simulink library "HVPS_AC120V_sfun_xk"  (R2022b)
settings: Solver=VariableStepAuto  StartTime=0.0  StopTime=10.0  RelTol=1e-3
Description:
  | Created by MapleSim.
settings Model: Creator=MapleSim  LastModifiedBy=BEDNASA

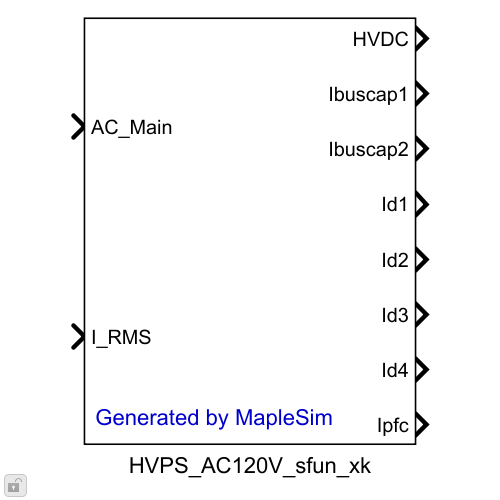
[thumbnail: Simulink's stored preview of the top-level diagram]
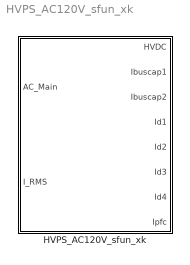
== system HVPS_AC120V_sfun_xk ==
  HVPS_AC120V_sfun_xk : Subsystem  Description=Subsystem: HVPS_AC120V_sfun_xk  mask(HVPS_AC120V_sfun_xk){ic=[186.676190233249, 186.676190233249, 0.], Par1=.1e-2, Par2=.83e-8, Par3=.5e-4, Par4=.1, Par5=.5e-2, Par6=.6, Par7=298.15, Par8=0., Par9=298.15, Par10=0., Par11=298.15, Par12=0., Par13=298.15, Par14=0., Par15=.1e-1, Par16=298.15, Par17=298.15, Par18=.1e8, Par19=298.15, Par20=298.15, Par21=298.15, Par22=298.15, Par23=.4041e-2, Par24=298.15, Par25=298.15, Par26=.4041e-2, Par27=298.15, Par28=298.15, Par29=1., Par30=1., Par31=.3e-2, Par32=.1e4, Par33=.625e-4, ExtData=, MinStep=1/40, TimeStep_Solver=1e-4}
      mask prompts: ic "Initial Conditions:"; Par1 "C_buscap:"; Par2 "G_off:"; Par3 "L_line:"; Par4 "R_buscap:"; Par5 "R_diode:"; Par6 "R_line:"; Par7 "ID1_T:"; Par8 "ID1_Vknee:"; Par9 "ID2_T:"; Par10 "ID2_Vknee:"; Par11 "ID3_T:"; Par12 "ID3_Vknee:"; Par13 "ID4_T:"; Par14 "ID4_Vknee:"; Par15 "R3_R:"; Par16 "R3_T_ref:"; Par17 "R3_T:"; Par18 "R4_R:"; Par19 "R4_T_ref:"; Par20 "R4_T:"; Par21 "R_BusCap1_T_ref:"; Par22 "R_BusCap1_T:"; Par23 "R_BusCap1_alpha:"; Par24 "R_BusCap2_T_ref:"; Par25 "R_BusCap2_T:"; Par26 "R_BusCap2_alpha:"; Par27 "R_Line_T_ref:"; Par28 "R_Line_T:"; Par29 "k1:"; Par30 "k2:"; Par31 "k:"; Par32 "Rising:"; Par33 "Td:"; ExtData "Extended Visualization Data - File Name (leave blank to disable):"; MinStep "Extended Visualization Data - Minimum Sample Step:"; TimeStep_Solver "Time Step - Solver:"
      mask help:
      | Variable Definitions
      |
      | Variable(s) in the Initial Condition Vector:
      |      x[ 0] = `Main.AC120V1.C_BusCap1.v`(t)
      |      x[ 1] = `Main.AC120V1.C_BusCap2.v`(t)
      |      x[ 2] = `Main.AC120V1.L_Line.i`(t)
      |
      | Variable(s) in the Output Vector:
      |    HVDC:
      |      y[ 0] = `Main.AC120V1.HVDC`(t)
      |    Ibuscap1:
      |      y[ 1] = `Main.AC120V1.Ibuscap1`(t)
      |    Ibuscap2:
      |      y[ 2] = `Main.AC120V1.Ibuscap2`(t)
      |    Id1:
      |      y[ 3] = `Main.AC120V1.Id1`(t)
      |    Id2:
      |      y[ 4] = `Main.AC120V1.Id2`(t)
      |    Id3:
      |      y[ 5] = `Main.AC120V1.Id3`(t)
      |    Id4:
      |      y[ 6] = `Main.AC120V1.Id4`(t)
      |    Ipfc:
      |      y[ 7] = `Main.AC120V1.Ipfc`(t)
      |
      | Variable(s) in the Input Vector:
      |    AC_Main:
      |      y[ 0] = `Main.AC120V1.AC_Main`(t)
      |    I_RMS:
      |      y[ 1] = `Main.AC120V1.I_RMS`(t)
      |
      | Parameter(s):
      |      p[ 0] = `Main.AC120V1.C_buscap` (default = .1e-2)
      |      p[ 1] = `Main.AC120V1.G_off` (default = .83e-8)
      |      p[ 2] = `Main.AC120V1.L_line` (default = .5e-4)
      |      p[ 3] = `Main.AC120V1.R_buscap` (default = .1)
      |      p[ 4] = `Main.AC120V1.R_diode` (default = .5e-2)
      |      p[ 5] = `Main.AC120V1.R_line` (default = .6)
      |      p[ 6] = `Main.AC120V1.ID1.T` (default = 298.15)
      |      p[ 7] = `Main.AC120V1.ID1.Vknee` (default = 0.)
      |      p[ 8] = `Main.AC120V1.ID2.T` (default = 298.15)
      |      p[ 9] = `Main.AC120V1.ID2.Vknee` (default = 0.)
      |      p[10] = `Main.AC120V1.ID3.T` (default = 298.15)
      |      p[11] = `Main.AC120V1.ID3.Vknee` (default = 0.)
      |      p[12] = `Main.AC120V1.ID4.T` (default = 298.15)
      |      p[13] = `Main.AC120V1.ID4.Vknee` (default = 0.)
      |      p[14] = `Main.AC120V1.R3.R` (default = .1e-1)
      |      p[15] = `Main.AC120V1.R3.T_ref` (default = 298.15)
      |      p[16] = `Main.AC120V1.R3.T` (default = 298.15)
      |      p[17] = `Main.AC120V1.R4.R` (default = .1e8)
      |      p[18] = `Main.AC120V1.R4.T_ref` (default = 298.15)
      |      p[19] = `Main.AC120V1.R4.T` (default = 298.15)
      |      p[20] = `Main.AC120V1.R_BusCap1.T_ref` (default = 298.15)
      |      p[21] = `Main.AC120V1.R_BusCap1.T` (default = 298.15)
      |      p[22] = `Main.AC120V1.R_BusCap1.alpha` (default = .4041e-2)
      |      p[23] = `Main.AC120V1.R_BusCap2.T_ref` (default = 298.15)
      |      p[24] = `Main.AC120V1.R_BusCap2.T` (default = 298.15)
      |      p[25] = `Main.AC120V1.R_BusCap2.alpha` (default = .4041e-2)
      |      p[26] = `Main.AC120V1.R_Line.T_ref` (default = 298.15)
      |      p[27] = `Main.AC120V1.R_Line.T` (default = 298.15)
      |      p[28] = `Main.AC120V1.add.k1` (default = 1.)
      |      p[29] = `Main.AC120V1.add.k2` (default = 1.)
      |      p[30] = `Main.AC120V1.const.k` (default = .3e-2)
      |      p[31] = `Main.AC120V1.slewRateLimiter.Rising` (default = .1e4)
      |      p[32] = `Main.AC120V1.slewRateLimiter.Td` (default = .625e-4)
      mask Help: <!DOCTYPE html PUBLIC "-//W3C//DTD HTML 4.01 Transitional//EN" "http://www.w3.org/TR/1999/REC-html401-19991224/loose.dtd"> <html lang="en"> <head> <title>HVPS_AC120V_sfun_xk :: MapleSim model</title> <style type="text/css"> body { background-color: white; margin:10px;} h1 { color: #990000; font-size: x-large; } h2 { color: #990000; font-size: large; margin-top:0ex;     margin-bottom:0ex;   font-weight:bold;  } h3 { color:#990000;  margin-top:0ex;   margin-bottom:0ex;  font-weight:bold;    font-size: medium; } h4 { color:black;    margin-top:0ex;   margin-bottom:0ex;  font-weight:bold;    font-size: medium; } /* Vertical space in tables other than the header and footer banners */ table.body { margin-top: 2ex; margin-bottom: 2ex;} /* Make the text shrink to fit narrow windows, but not stretch too far in wide windows. */ p,h1,h2,div.content div { max-width: 600px; } pre.codeinput { background: #EEEEEE; padding: 10px;} @media print { pre.codeinput { word-wrap:break-word; width:100%; } } span.keyword { color: #0000FF} span.comment { color: #228B22} span.string { color: #A020F0} span.untermstring {color: #B20000} span.syscmd { color: #B28C00} pre.error { color: red;} p.footer { text-align: right; font-size: xx-small; font-weight: lighter; font-style: italic; color: gray; } </style> <meta name="generator" content="DocBook XSL Stylesheets V1.52.2"> <meta name="chunktype" content="refpage"> <meta http-equiv="Content-Script-Type" content="text/javascript"> </head> <body> <a name="top_of_page"></a> <p style="font-size:1px;"> <a name="f8-894621"></a> <a name="transferfcn"></a> <a class="indexterm" name="zmw57dd0e42758"></a></p> <h1 class="reftitle">HVPS_AC120V_sfun_xk</h1> <p>Simulink Block generated by MapleSim Connector</p> <p><a name="f8-894627"></a></p> <h1>Description <span class="inlinemediaobject"></span></h1> <p><a class="indexterm" name="zmw57dd0e42781"></a></p> <p>The HVPS_AC120V_sfun_xk model runs in the continuous domain and is created in the MapleSim modeling environment. The discrete S-Function block HVPS_AC120V_sfun_xk is created using MapleSim Connector. The block is a 2-input, 8-output, 33-parameter system.</p> <p><a name="f8-894641"></a></p> <h1>System Variables</h1> <p>The following variables are used in the S-Function block:</p>  State Variable(s)<dl><dd>x[ 0] = `Main.AC120V1.C_BusCap1.v`(t)</dd></br><dd>x[ 1] = `Main.AC120V1.C_BusCap2.v`(t)</dd></br><dd>x[ 2] = `Main.AC120V1.L_Line.i`(t)</dd></br><dd>x[ 3] = `Main.AC120V1.slewRateLimiter.y`(t)   (*)</dd></br></dl><p>(*) fixed initial condition due to initial equation</p> Output Variable(s)<dl><dd>HVDC:</dd></br><dd>&nbsp;&nbsp;y[ 0] = `Main.AC120V1.HVDC`(t)</dd></br><dd>Ibuscap1:</dd></br><dd>&nbsp;&nbsp;y[ 1] = `Main.AC120V1.Ibuscap1`(t)</dd></br><dd>Ibuscap2:</dd></br><dd>&nbsp;&nbsp;y[ 2] = `Main.AC120V1.Ibuscap2`(t)</dd></br><dd>Id1:</dd></br><dd>&nbsp;&nbsp;y[ 3] = `Main.AC120V1.Id1`(t)</dd></br><dd>Id2:</dd></br><dd>&nbsp;&nbsp;y[ 4] = `Main.AC120V1.Id2`(t)</dd></br><dd>Id3:</dd></br><dd>&nbsp;&nbsp;y[ 5] = `Main.AC120V1.Id3`(t)</dd></br><dd>Id4:</dd></br><dd>&nbsp;&nbsp;y[ 6] = `Main.AC120V1.Id4`(t)</dd></br><dd>Ipfc:</dd></br><dd>&nbsp;&nbsp;y[ 7] = `Main.AC120V1.Ipfc`(t)</dd></br></dl> Input Variable(s)<dl><dd>AC_Main:</dd></br><dd>&nbsp;&nbsp;y[ 0] = `Main.AC120V1.AC_Main`(t)</dd></br><dd>I_RMS:</dd></br><dd>&nbsp;&nbsp;y[ 1] = `Main.AC120V1.I_RMS`(t)</dd></br></dl> Parameter(s)<dl><dd>p[ 0] = `Main.AC120V1.C_buscap` (default = .1e-2)</dd></br><dd>p[ 1] = `Main.AC120V1.G_off` (default = .83e-8)</dd></br><dd>p[ 2] = `Main.AC120V1.L_line` (default = .5e-4)</dd></br><dd>p[ 3] = `Main.AC120V1.R_buscap` (default = .1)</dd></br><dd>p[ 4] = `Main.AC120V1.R_diode` (default = .5e-2)</dd></br><dd>p[ 5] = `Main.AC120V1.R_line` (default = .6)</dd></br><dd>p[ 6] = `Main.AC120V1.ID1.T` (default = 298.15)</dd></br><dd>p[ 7] = `Main.AC120V1.ID1.Vknee` (default = 0.)</dd></br><dd>p[ 8] = `Main.AC120V1.ID2.T` (default = 298.15)</dd></br><dd>p[ 9] = `Main.AC120V1.ID2.Vknee` (default = 0.)</dd></br><dd>p[10] = `Main.AC120V1.ID3.T` (default = 298.15)</dd></br><dd>p[11] = `Main.AC120V1.ID3.Vknee` (default = 0.)</dd></br><dd>p[12] = `Main.AC120V1.ID4.T` (default = 298.15)</dd></br><dd>p[13] = `Main.AC120V1.ID4.Vknee` (default = 0.)</dd></br><dd>p[14] = `Main.AC120V1.R3.R` (default = .1e-1)</dd></br><dd>p[15] = `Main.AC120V1.R3.T_ref` (default = 298.15)</dd></br><dd>p[16] = `Main.AC120V1.R3.T` (default = 298.15)</dd></br><dd>p[17] = `Main.AC120V1.R4.R` (default = .1e8)</dd></br><dd>p[18] = `Main.AC120V1.R4.T_ref` (default = 298.15)</dd></br><dd>p[19] = `Main.AC120V1.R4.T` (default = 298.15)</dd></br><dd>p[20] = `Main.AC120V1.R_BusCap1.T_ref` (default = 298.15)</dd></br><dd>p[21] = `Main.AC120V1.R_BusCap1.T` (default = 298.15)</dd></br><dd>p[22] = `Main.AC120V1.R_BusCap1.alpha` (default = .4041e-2)</dd></br><dd>p[23] = `Main.AC120V1.R_BusCap2.T_ref` (default = 298.15)</dd></br><dd>p[24] = `Main.AC120V1.R_BusCap2.T` (default = 298.15)</dd></br><dd>p[25] = `Main.AC120V1.R_BusCap2.alpha` (default = .4041e-2)</dd></br><dd>p[26] = `Main.AC120V1.R_Line.T_ref` (default = 298.15)</dd></br><dd>p[27] = `Main.AC120V1.R_Line.T` (default = 298.15)</dd></br><dd>p[28] = `Main.AC120V1.add.k1` (default = 1.)</dd></br><dd>p[29] = `Main.AC120V1.add.k2` (default = 1.)</dd></br><dd>p[30] = `Main.AC120V1.const.k` (default = .3e-2)</dd></br><dd>p[31] = `Main.AC120V1.slewRateLimiter.Rising` (default = .1e4)</dd></br><dd>p[32] = `Main.AC120V1.slewRateLimiter.Td` (default = .625e-4)</dd></br></dl></p> <p><a name="f8-894651"></a></p><h1>Data Type Support</h1> <p>The HVPS_AC120V_sfun_xk block accepts inputs and outputs signals of type <tt>double</tt>.</p> <a name="f8-894653"></a><h1>Parameters</h1><dl> <dt><a name="zmw57dd0e42948"></a><b><span class="term">Initial Condition</span>s</b></dt> <dd> <p>The row vector of initial conditions. A vector can be specified to initialize the state variables of the system.</p></dd> <dd> <p>The initial values of the following states are fixed based upon initial equations: x[ 3]</p></dd><dt><a name="zmw57dd0e42958"></a><span class="term"><b>Parameters</b></span></dt> <dd> <p>The scalars or the row vector of tunable parameters.</p></dd> </dl> <dt><a name="zmw57dd0e42968"></a> </dt><h1>Characteristics</h1> <table cellspacing="0" class="body" cellpadding="4" border="2"><colgroup><col width="41%"><col width="59%"></colgroup><tbody> <tr valign="top"><td bgcolor="#F2F2F2"><p>Direct Feedthrough</p></td><td bgcolor="#F2F2F2"><p>Yes, only if the block has no state variables.</p></td></tr> <tr valign="top"><td bgcolor="#F2F2F2"><p>Sample Time</p></td><td bgcolor="#F2F2F2"><p> Discrete</p></td></tr> <tr valign="top"><td bgcolor="#F2F2F2"><p>Scalar Expansion</p></td><td bgcolor="#F2F2F2"><p>No</p></td></tr> <tr valign="top"><td bgcolor="#F2F2F2"><p>State</p></td><td bgcolor="#F2F2F2"><p>Yes</p></td></tr> <tr valign="top"><td bgcolor="#F2F2F2"><p>Dimensionalized</p></td><td bgcolor="#F2F2F2"><p>Yes</p></td></tr> <tr valign="top"><td bgcolor="#F2F2F2"><p>Zero Crossing</p></td><td bgcolor="#F2F2F2"><p>Yes</p></td></tr> </tbody></table> <p></p><h1>Maple / MapleSim / MapleSim Connector Details</h1> <p></p><dd><p>Maple 2021.1, X86 64 WINDOWS, May 19 2021, Build ID 1539851</p></dd><dd><p>MapleSim 2021.1 Control Design, Wed May 19 23:38:09 EDT 2021, 1539851</p></dd><dd><p>MapleSim 2021.1 Connector for FMI, Wed May 19 23:38:47 EDT 2021, 1539851</p></dd><dd><p>GlobalOptimization 2021.0, Thu Mar 11 13:21:11 EST 2021, 1524228</p></dd><dd><p>MapleSim 2021.1, Wed May 19 23:37:53 EDT 2021, 1539851</p></dd><dd><p>MapleSim 2021.1 Connector, Wed May 19 23:39:01 EDT 2021, 1539851</p></dd><p></p></body></html>
      mask Display: color('blue');text(5,12,'Generated by MapleSim');

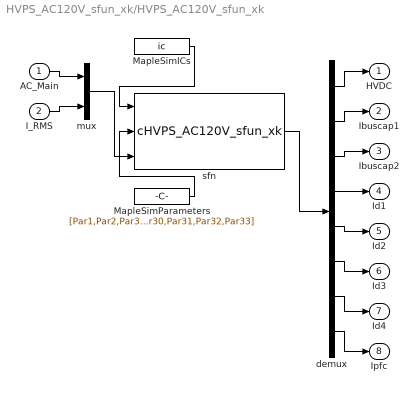
== system HVPS_AC120V_sfun_xk/HVPS_AC120V_sfun_xk ==
  AC_Main : Inport
  I_RMS : Inport  Port=2
  MapleSimICs : Constant  Value=ic
  MapleSimParameters : Constant  Value=[Par1,Par2,Par3,Par4,Par5,Par6,Par7,Par8,Par9,Par10,Par11,Par12,Par13,Par14,Par15,Par16,Par17,Par18,Par19,Par20,Par21,Par22,Par23,Par24,Par25,Par26,Par27,Par28,Par29,Par30,Par31,Par32,Par33]
  demux : Demux  Outputs=[1 1 1 1 1 1 1 1]
  mux : Mux  Inputs=2
  sfn : S-Function  Description=Generated by MapleSim  FunctionName=cHVPS_AC120V_sfun_xk  Parameters=ExtData,MinStep,TimeStep_Solver  PortCounts=[3, 1]  SFunctionDeploymentMode=off  EnableBusSupport=off
  HVDC : Outport
  Ibuscap1 : Outport  Port=2
  Ibuscap2 : Outport  Port=3
  Id1 : Outport  Port=4
  Id2 : Outport  Port=5
  Id3 : Outport  Port=6
  Id4 : Outport  Port=7
  Ipfc : Outport  Port=8
  wires:
  MapleSimICs/1 -> sfn/1
  MapleSimParameters/1 -> sfn/2
  mux/1 -> sfn/3
  AC_Main/1 -> mux/1
  I_RMS/1 -> mux/2
  sfn/1 -> demux/1
  demux/1 -> HVDC/1
  demux/2 -> Ibuscap1/1
  demux/3 -> Ibuscap2/1
  demux/4 -> Id1/1
  demux/5 -> Id2/1
  demux/6 -> Id3/1
  demux/7 -> Id4/1
  demux/8 -> Ipfc/1
